simulink model "State_Based_Output_Feedback_Controller_2"  (R2020b)
settings: Solver=ode45  StartTime=0.0  StopTime=4  MaxStep=0.08  RelTol=1e-3
libraries: pid_lib x1
settings Model: Creator=Kevin  LastModifiedBy=francesco

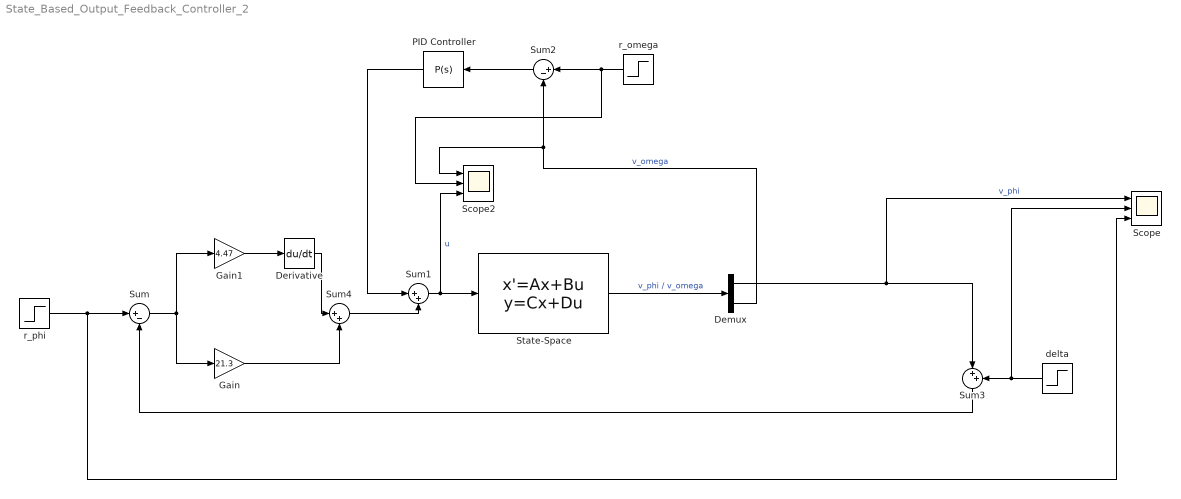
== system State_Based_Output_Feedback_Controller_2 ==
  Demux : Demux  Outputs=2
  Derivative : Derivative
  Gain : Gain  Gain=21.3
  Gain1 : Gain  Gain=4.47
  PID Controller : pid_lib/PID Controller  Controller=P  Form=Parallel  TimeDomain=Continuous-time  UseExternalTs=off  SampleTime=-1  IntegratorMethod=Forward Euler  FilterMethod=Forward Euler  ControllerParametersSource=internal  P=2.31  I=1  D=0  UseFilter=on  N=100  TunerSelectOption=Transfer Function Based (PID Tuner App)  InitialConditionSource=internal  InitialConditionForIntegrator=0  InitialConditionForFilter=0  DifferentiatorICPrevScaledInput=0  ExternalReset=none  TrackingMode=off  Kt=1  LimitOutput=off  SatLimitsSource=internal  UpperSaturationLimit=inf  LowerSaturationLimit=-inf  LinearizeAsGain=on  AntiWindupMode=none  Kb=1  POutMin=[]  POutMax=[]  IOutMin=[]  IOutMax=[]  DOutMin=[]  DOutMax=[]  NOutMin=[]  NOutMax=[]  SumOutMin=[]  SumOutMax=[]  SaturationOutMin=[]  SaturationOutMax=[]  PParamMin=[]  PParamMax=[]  IParamMin=[]  IParamMax=[]  DParamMin=[]  DParamMax=[]  NParamMin=[]  NParamMax=[]  KbParamMin=[]  KbParamMax=[]  KtParamMin=[]  KtParamMax=[]  KbOutMin=[]  KbOutMax=[]  KtOutMin=[]  KtOutMax=[]  IntegratorOutMin=[]  IntegratorOutMax=[]  FilterOutMin=[]  FilterOutMax=[]  SumI1OutMin=[]  SumI1OutMax=[]  SumI2OutMin=[]  SumI2OutMax=[]  SumI3OutMin=[]  SumI3OutMax=[]  SumI4OutMin=[]  SumI4OutMax=[]  SumDOutMin=[]  SumDOutMax=[]  DifferentiatorOutMin=[]  DifferentiatorOutMax=[]  FilterDiffOutCoefMin=[]  FilterDiffOutCoefMax=[]  ReciprocalOutMin=[]  ReciprocalOutMax=[]  SumDenOutMin=[]  SumDenOutMax=[]  SumNumOutMin=[]  SumNumOutMax=[]  DivideOutMin=[]  DivideOutMax=[]  UdiffTsProdOutMin=[]  UdiffTsProdOutMax=[]  NTsProdOutMin=[]  NTsProdOutMax=[]  UintegralTsProdOutMin=[]  UintegralTsProdOutMax=[]  UngainTsProdOutMin=[]  UngainTsProdOutMax=[]  IntegratorContinuousStateAttributes=''  IntegratorStateMustResolveToSignalObject=off  IntegratorRTWStateStorageClass=Auto  FilterContinuousStateAttributes=''  FilterStateMustResolveToSignalObject=off  FilterRTWStateStorageClass=Auto  ParallelPVariant=InternalParameters  IdealPVariant=Disabled  IVariant=Disabled  DVariant=Disabled  IntegratorVariant=Disabled  SatVariant=Disabled  AWVariant=Disabled  PCopyVariant=Disabled  TRVariant=Disabled  FdbkBlocksVariant=Forward  IdealPFdbkVariant=Disabled  SatFdbkVariant=Disabled  DerivativeFilterVariant=Disabled  NVariant=Disabled  NCopyVariant=Disabled_SignalSpec  FilterICVariant=Disabled  IntegratorICVariant=Disabled  ExternalResetVariant=Disabled  TRSumVariant=Passthrough  SumFdbkVariant=Disabled  SumVariant=Passthrough_P  TsampFilterVariant=InternalTs  TsampNgainVariant=Passthrough  TsampIntegralVariant=Disabled_SignalSpec  ExternalSaturationOutDataTypeStr=Inherit: Same as second input
  Scope : Scope  NumInputPorts=3
  Scope2 : Scope  NumInputPorts=3
  State-Space : StateSpace  A=[0 1 0; 23.5031 0 0.0045; -23.5031 0 -19.9513]  B=[0; 0.1393; -621.6819]  C=[107.47 0 0; 0 0 1/30]  D=[0; 0]  InitialCondition=[0.0019 0 0]
  Sum : Sum  Inputs=|+-
  Sum1 : Sum  Inputs=|++
  Sum2 : Sum  Inputs=|+-
  Sum3 : Sum  Inputs=|++
  Sum4 : Sum  Inputs=|++
  delta : Step  Time=1.5  After=0.2  SampleTime=0
  r_omega : Step  Time=2.5  After=2.5  SampleTime=0
  r_phi : Step  Time=0  After=0  SampleTime=0
  wires:
  Sum/1 -> Gain1/1, Gain/1
  Sum1/1 -> Scope2/3, State-Space/1  "u"
  r_omega/1 -> Scope2/2, Sum2/1
  State-Space/1 -> Demux/1  "v_phi / v_omega"
  Demux/2 -> Sum2/2, Scope2/1  "v_omega"
  Demux/1 -> Scope/1, Sum3/1  "v_phi"
  delta/1 -> Scope/2, Sum3/2
  Sum3/1 -> Sum/2
  r_phi/1 -> Sum/1, Scope/3
  Sum2/1 -> PID Controller/1
  PID Controller/1 -> Sum1/1
  Gain/1 -> Sum4/2
  Gain1/1 -> Derivative/1
  Derivative/1 -> Sum4/1
  Sum4/1 -> Sum1/2
